simulink subsystem "Closed"  (R2023b)
settings: Solver=VariableStepAuto  StartTime=0.0  StopTime=10.0  RelTol=1e-3
libraries: simulink x5
settings Model: Creator=diego  LastModifiedBy=rebek

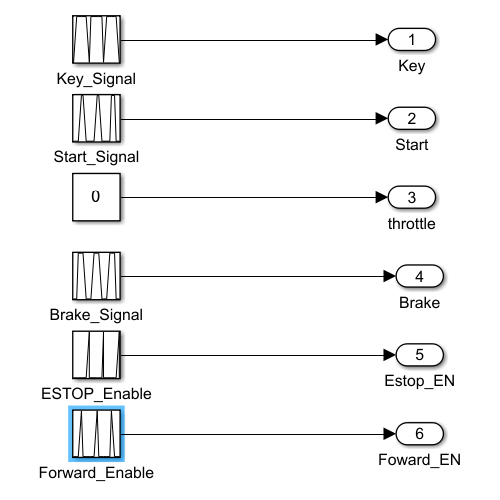
[thumbnail: Simulink's stored preview of the top-level diagram]
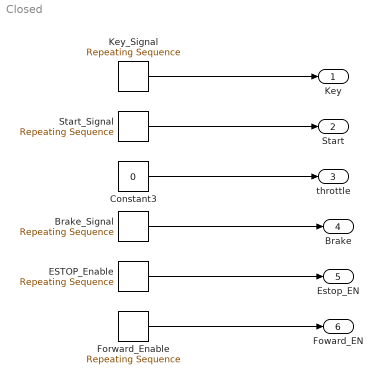
== system Closed ==
  Brake_Signal : simulink/Sources/Repeating Sequence  rep_seq_t=[0 100 200 300 400 500 600]  rep_seq_y=[0 0 1 1 1 0 0]
  Constant3 : Constant  Value=0
  ESTOP_Enable : simulink/Sources/Repeating Sequence  rep_seq_t=[0 100 200 300 400 500 600]  rep_seq_y=[0 0 0 0 0 0 1]
  Forward_Enable : simulink/Sources/Repeating Sequence  rep_seq_t=[0 100 200 300 400 500 600]  rep_seq_y=[0 0 0 1 0 0 0]
  Key_Signal : simulink/Sources/Repeating Sequence  rep_seq_t=[0 100 200 300 400 500 600]  rep_seq_y=[0 1 1 1 1 1 0]
  Start_Signal : simulink/Sources/Repeating Sequence  rep_seq_t=[0 100 200 300 400 500 600]  rep_seq_y=[0 0 0 1 1 0 0]
  Key : Outport
  Start : Outport  Port=2
  throttle : Outport  Port=3
  Brake : Outport  Port=4
  Estop_EN : Outport  Port=5
  Foward_EN : Outport  Port=6
  wires:
  Constant3/1 -> throttle/1
  Brake_Signal/1 -> Brake/1
  Start_Signal/1 -> Start/1
  Key_Signal/1 -> Key/1
  ESTOP_Enable/1 -> Estop_EN/1
  Forward_Enable/1 -> Foward_EN/1
